simulink model "LGS_allFaultStuffDeleted"  (R2019b)
settings: Solver=FixedStepDiscrete  StartTime=0.0  StopTime=45.0  FixedStep=0.1  RelTol=1e-3
model workspace (MAT data in the model file):
  fipData : object (value not decoded)
  fipName : object (value not decoded)
  stepSize = 0.1
libraries: commrandsrc3 x16, simulink x3, LibFailureCondition x1
(part 6 of 7)

== stateflow chart LGS_allFaultStuffDeleted/Digital Part/Computing module2/GenericMonitoring9/GenericMonitoring2 ==
  state SensorValid
    entry: anomaly = false;
  state Channel1Invalid
  state SensorInvalid
    entry: anomaly = true;
  note: If at t the three channels are considered as valid and are equal, then the
      | value considered by the control software is this common value.
  state Channel2Invalid
  note: If a channel has been eliminated previously, and if at t the two remaining
      | channels are not equal, then the sensor is definitely considered as invalid.
  state Channel3Invalid
  note: If at t one channel is different from the two others for the first time (i.e.,
      | the three channels were considered as valid up to t), then this channel is
      | considered as invalid and is definitely eliminated. Only the two remaining
      | channels are considered in the future. At time t, the value considered by the
      | control software is the common value of the two remaining channels.
  (default) -> SensorValid
  SensorValid -> Channel1Invalid [order 1] : [(((Channel3&&Channel2) || ((~Channel3)&&(~Channel2))) && ((Channel1 && (~Channel2)) || ((~Channel1) && Channel2)))]
  Channel1Invalid -> SensorInvalid : [((Channel2 && (~Channel3)) || ((~Channel2) && Channel3))]
  SensorValid -> Channel2Invalid [order 2] : [(((Channel1&&Channel3) || ((~Channel1)&&(~Channel3))) && ((Channel1 && (~Channel2)) || ((~Channel1) && Channel2)))]
  SensorValid -> Channel3Invalid [order 3] : [(((Channel1&&Channel2) || ((~Channel1)&&(~Channel2))) && ((Channel1 && (~Channel3)) || ((~Channel1) && Channel3)))]
  Channel2Invalid -> SensorInvalid : [((Channel1 && (~Channel3)) || ((~Channel1) && Channel3))]
  Channel3Invalid -> SensorInvalid : [((Channel2 && (~Channel1)) || ((~Channel2) && Channel1))]
  data: Channel1 input boolean; Channel2 input boolean; Channel3 input boolean; anomaly output boolean

== stateflow chart LGS_allFaultStuffDeleted/Doors/EV close doors/EV close doors ==
  state state_EVCloseDoorsOpened
    en: EVCloseDoorsPresure_out = false;
  state state_EVCloseDoorsClose
    en: EVCloseDoorsPresure_out = false;
  state state_EVCloseDoorsClosed
    en: EVCloseDoorsPresure_out = true;
  (default) -> state_EVCloseDoorsOpened
  state_EVCloseDoorsClosed -> state_EVCloseDoorsOpened : [((~signal_in) || (~EVCloseDoorsPresure_in)) && ~fail]
  state_EVCloseDoorsOpened -> state_EVCloseDoorsClose : [(signal_in && EVCloseDoorsPresure_in && ~fail)]
  state_EVCloseDoorsClose -> state_EVCloseDoorsOpened [order 2] : [((~signal_in) || (~EVCloseDoorsPresure_in)) && ~fail]
  state_EVCloseDoorsClose -> state_EVCloseDoorsClosed [order 1] : [(signal_in && EVCloseDoorsPresure_in && ~fail)]
  data: signal_in input boolean; EVCloseDoorsPresure_in input boolean [0..1]; EVCloseDoorsPresure_out output boolean [0..1]; fail input

== stateflow chart LGS_allFaultStuffDeleted/Doors/EV open doors/EV open doors ==
  state state_EVOpenDoorsOpened
    en: EVOpenDoorsPresure_out = false;
  state state_EVOpenDoorsClose
    en: EVOpenDoorsPresure_out = false;
  state state_EVOpenDoorsClosed
    en: EVOpenDoorsPresure_out = true;
  (default) -> state_EVOpenDoorsOpened
  state_EVOpenDoorsClosed -> state_EVOpenDoorsOpened : [((~signal_in) || (~EVOpenDoorsPresure_in)) && ~fail]
  state_EVOpenDoorsOpened -> state_EVOpenDoorsClose : [(signal_in && EVOpenDoorsPresure_in && ~fail)]
  state_EVOpenDoorsClose -> state_EVOpenDoorsOpened [order 2] : [((~signal_in) || (~EVOpenDoorsPresure_in)) && ~fail]
  state_EVOpenDoorsClose -> state_EVOpenDoorsClosed [order 1] : [(signal_in && EVOpenDoorsPresure_in && ~fail)]
  data: signal_in input boolean; EVOpenDoorsPresure_in input boolean [0..1]; EVOpenDoorsPresure_out output boolean [0..1]; fail input

== stateflow chart LGS_allFaultStuffDeleted/Doors/left door zylinder/door zylinder ==
  state state_DoorZylinderClosedLocked
    en: doorZylinderOpen = false;
    en: doorZylinderLockedClosed = true;
  state state_DoorZylinderClosedLock
    en: doorZylinderOpen = false;
    en: doorZylinderLockedClosed = false;
  state state_DoorZylinderClose
    en: doorZylinderOpen = false;
    en: doorZylinderLockedClosed = false;
    en: time = int8(1);
    du: time = time - 1;
  state state_DoorZylinderClosedLockingPaused
    en: doorZylinderOpen = false;
    en: doorZylinderLockedClosed = false;
  state state_DoorZylinderClosedUnlock
    en: doorZylinderOpen = false;
    en: doorZylinderLockedClosed = false;
  state state_DoorZylinderMovingPaused
    en: doorZylinderOpen = false;
    en: doorZylinderLockedClosed = false;
  state state_DoorZylinderOpen
    en: doorZylinderOpen = false;
    en: doorZylinderLockedClosed = false;
    en: time = int8(1);
    du: time = time - 1;
  state state_DoorZylinderOpened
    en: doorZylinderOpen = true;
    en: doorZylinderLockedClosed = false;
  state state_DoorZylinderOpenedPaused
    en: doorZylinderOpen = false;
    en: doorZylinderLockedClosed = false;
  (default) -> state_DoorZylinderClosedLocked
  state_DoorZylinderClose -> state_DoorZylinderClosedLock [order 1] : [((time==0) && (~presureOpenDoor) && presureCloseDoor && (~fail))]
  state_DoorZylinderClosedLock -> state_DoorZylinderClosedLocked [order 1] : [((~presureOpenDoor) && presureCloseDoor && (~fail))]
  state_DoorZylinderClosedUnlock -> state_DoorZylinderClosedLock [order 1] : [((~presureOpenDoor) && presureCloseDoor && (~fail))]
  state_DoorZylinderClosedLock -> state_DoorZylinderClosedUnlock [order 2] : [(presureOpenDoor && (~presureCloseDoor) && (~fail))]
  state_DoorZylinderClosedLocked -> state_DoorZylinderClosedUnlock : [(presureOpenDoor && (~presureCloseDoor) && (~fail))]
  state_DoorZylinderClosedLockingPaused -> state_DoorZylinderClosedLock [order 2] : [((~presureOpenDoor) && presureCloseDoor && (~fail))]
  state_DoorZylinderClosedLock -> state_DoorZylinderClosedLockingPaused [order 3] : [(((~presureOpenDoor) && (~presureCloseDoor)) || (presureOpenDoor && presureCloseDoor) || fail)]
  state_DoorZylinderClose -> state_DoorZylinderMovingPaused [order 3] : [(((~presureOpenDoor) && (~presureCloseDoor)) || (presureOpenDoor && presureCloseDoor) || fail)]
  state_DoorZylinderOpenedPaused -> state_DoorZylinderClose [order 2] : [((~presureOpenDoor) && presureCloseDoor && (~fail))]
  state_DoorZylinderOpen -> state_DoorZylinderClose [order 2] : [((~presureOpenDoor) && presureCloseDoor && (~fail))]
  state_DoorZylinderClose -> state_DoorZylinderOpen [order 2] : [(presureOpenDoor && (~presureCloseDoor) && (~fail))]
  state_DoorZylinderMovingPaused -> state_DoorZylinderClose [order 2] : [((~presureOpenDoor) && presureCloseDoor && (~fail))]
  state_DoorZylinderOpened -> state_DoorZylinderClose [order 2] : [((~presureOpenDoor) && presureCloseDoor && (~fail))]
  state_DoorZylinderClosedLockingPaused -> state_DoorZylinderClosedUnlock [order 1] : [(presureOpenDoor && (~presureCloseDoor) && (~fail))]
  state_DoorZylinderClosedUnlock -> state_DoorZylinderClosedLockingPaused [order 2] : [(((~presureOpenDoor) && (~presureCloseDoor)) || (presureOpenDoor && presureCloseDoor) || fail)]
  state_DoorZylinderClosedUnlock -> state_DoorZylinderOpen [order 3] : [(presureOpenDoor && (~presureCloseDoor) && (~fail))]
  state_DoorZylinderOpen -> state_DoorZylinderMovingPaused [order 3] : [(((~presureOpenDoor) && (~presureCloseDoor)) || (presureOpenDoor && presureCloseDoor) || fail)]
  state_DoorZylinderMovingPaused -> state_DoorZylinderOpen [order 1] : [(presureOpenDoor && (~presureCloseDoor) && (~fail))]
  state_DoorZylinderOpen -> state_DoorZylinderOpened [order 1] : [((time==0) && presureOpenDoor && (~presureCloseDoor) && (~fail))]
  state_DoorZylinderOpened -> state_DoorZylinderOpenedPaused [order 1] : [(((~presureOpenDoor) && (~presureCloseDoor) && (~fail)) || (presureOpenDoor && presureCloseDoor && (~fail)))]
  state_DoorZylinderOpenedPaused -> state_DoorZylinderOpened [order 1] : [(presureOpenDoor && (~presureCloseDoor) && (~fail))]
  data: presureOpenDoor input boolean [0..1]; presureCloseDoor input boolean [0..1]; time local int8 [0..1]; doorZylinderLockedClosed output boolean; doorZylinderOpen output boolean; fail input boolean

== stateflow chart LGS_allFaultStuffDeleted/Doors/right door zylinder/door zylinder ==
  state state_DoorZylinderClosedLocked
    en: doorZylinderOpen = false;
    en: doorZylinderLockedClosed = true;
  state state_DoorZylinderClosedLock
    en: doorZylinderOpen = false;
    en: doorZylinderLockedClosed = false;
  state state_DoorZylinderClose
    en: doorZylinderOpen = false;
    en: doorZylinderLockedClosed = false;
    en: time = int8(1);
    du: time = time - 1;
  state state_DoorZylinderClosedLockingPaused
    en: doorZylinderOpen = false;
    en: doorZylinderLockedClosed = false;
  state state_DoorZylinderClosedUnlock
    en: doorZylinderOpen = false;
    en: doorZylinderLockedClosed = false;
  state state_DoorZylinderMovingPaused
    en: doorZylinderOpen = false;
    en: doorZylinderLockedClosed = false;
  state state_DoorZylinderOpen
    en: doorZylinderOpen = false;
    en: doorZylinderLockedClosed = false;
    en: time = int8(1);
    du: time = time - 1;
  state state_DoorZylinderOpened
    en: doorZylinderOpen = true;
    en: doorZylinderLockedClosed = false;
  state state_DoorZylinderOpenedPaused
    en: doorZylinderOpen = false;
    en: doorZylinderLockedClosed = false;
  (default) -> state_DoorZylinderClosedLocked
  state_DoorZylinderClose -> state_DoorZylinderClosedLock [order 1] : [((time==0) && (~presureOpenDoor) && presureCloseDoor && (~fail))]
  state_DoorZylinderClosedLock -> state_DoorZylinderClosedLocked [order 1] : [((~presureOpenDoor) && presureCloseDoor && (~fail))]
  state_DoorZylinderClosedUnlock -> state_DoorZylinderClosedLock [order 1] : [((~presureOpenDoor) && presureCloseDoor && (~fail))]
  state_DoorZylinderClosedLock -> state_DoorZylinderClosedUnlock [order 2] : [(presureOpenDoor && (~presureCloseDoor) && (~fail))]
  state_DoorZylinderClosedLocked -> state_DoorZylinderClosedUnlock : [(presureOpenDoor && (~presureCloseDoor) && (~fail))]
  state_DoorZylinderClosedLockingPaused -> state_DoorZylinderClosedLock [order 2] : [((~presureOpenDoor) && presureCloseDoor && (~fail))]
  state_DoorZylinderClosedLock -> state_DoorZylinderClosedLockingPaused [order 3] : [(((~presureOpenDoor) && (~presureCloseDoor)) || (presureOpenDoor && presureCloseDoor) || fail)]
  state_DoorZylinderClose -> state_DoorZylinderMovingPaused [order 3] : [(((~presureOpenDoor) && (~presureCloseDoor)) || (presureOpenDoor && presureCloseDoor) || fail)]
  state_DoorZylinderOpenedPaused -> state_DoorZylinderClose [order 2] : [((~presureOpenDoor) && presureCloseDoor && (~fail))]
  state_DoorZylinderOpen -> state_DoorZylinderClose [order 2] : [((~presureOpenDoor) && presureCloseDoor && (~fail))]
  state_DoorZylinderClose -> state_DoorZylinderOpen [order 2] : [(presureOpenDoor && (~presureCloseDoor) && (~fail))]
  state_DoorZylinderMovingPaused -> state_DoorZylinderClose [order 2] : [((~presureOpenDoor) && presureCloseDoor && (~fail))]
  state_DoorZylinderOpened -> state_DoorZylinderClose [order 2] : [((~presureOpenDoor) && presureCloseDoor && (~fail))]
  state_DoorZylinderClosedLockingPaused -> state_DoorZylinderClosedUnlock [order 1] : [(presureOpenDoor && (~presureCloseDoor) && (~fail))]
  state_DoorZylinderClosedUnlock -> state_DoorZylinderClosedLockingPaused [order 2] : [(((~presureOpenDoor) && (~presureCloseDoor)) || (presureOpenDoor && presureCloseDoor) || fail)]
  state_DoorZylinderClosedUnlock -> state_DoorZylinderOpen [order 3] : [(presureOpenDoor && (~presureCloseDoor) && (~fail))]
  state_DoorZylinderOpen -> state_DoorZylinderMovingPaused [order 3] : [(((~presureOpenDoor) && (~presureCloseDoor)) || (presureOpenDoor && presureCloseDoor) || fail)]
  state_DoorZylinderMovingPaused -> state_DoorZylinderOpen [order 1] : [(presureOpenDoor && (~presureCloseDoor) && (~fail))]
  state_DoorZylinderOpen -> state_DoorZylinderOpened [order 1] : [((time==0) && presureOpenDoor && (~presureCloseDoor) && (~fail))]
  state_DoorZylinderOpened -> state_DoorZylinderOpenedPaused [order 1] : [(((~presureOpenDoor) && (~presureCloseDoor) && (~fail)) || (presureOpenDoor && presureCloseDoor && (~fail)))]
  state_DoorZylinderOpenedPaused -> state_DoorZylinderOpened [order 1] : [(presureOpenDoor && (~presureCloseDoor) && (~fail))]
  data: presureOpenDoor input boolean [0..1]; presureCloseDoor input boolean [0..1]; time local int8 [0..1]; doorZylinderLockedClosed output boolean; doorZylinderOpen output boolean; fail input boolean

== stateflow chart LGS_allFaultStuffDeleted/Doors/front door zylinder/door cylinder ==
  state state_DoorZylinderClosedLocked
    en: doorZylinderOpen = false;
    en: doorZylinderLockedClosed = true;
  state state_DoorZylinderClosedLock
    en: doorZylinderOpen = false;
    en: doorZylinderLockedClosed = false;
  state state_DoorZylinderClose
    en: doorZylinderOpen = false;
    en: doorZylinderLockedClosed = false;
    en: time = int8(1);
    du: time = time - 1;
  state state_DoorZylinderClosedLockingPaused
    en: doorZylinderOpen = false;
    en: doorZylinderLockedClosed = false;
  state state_DoorZylinderClosedUnlock
    en: doorZylinderOpen = false;
    en: doorZylinderLockedClosed = false;
  state state_DoorZylinderMovingPaused
    en: doorZylinderOpen = false;
    en: doorZylinderLockedClosed = false;
  state state_DoorZylinderOpen
    en: doorZylinderOpen = false;
    en: doorZylinderLockedClosed = false;
    en: time = int8(1);
    du: time = time - 1;
  state state_DoorZylinderOpened
    en: doorZylinderOpen = true;
    en: doorZylinderLockedClosed = false;
  state state_DoorZylinderOpenedPaused
    en: doorZylinderOpen = false;
    en: doorZylinderLockedClosed = false;
  (default) -> state_DoorZylinderClosedLocked
  state_DoorZylinderClose -> state_DoorZylinderClosedLock [order 1] : [((time==0) && (~presureOpenDoor) && presureCloseDoor && (~fail))]
  state_DoorZylinderClosedLock -> state_DoorZylinderClosedLocked [order 1] : [((~presureOpenDoor) && presureCloseDoor && (~fail))]
  state_DoorZylinderClosedUnlock -> state_DoorZylinderClosedLock [order 1] : [((~presureOpenDoor) && presureCloseDoor && (~fail))]
  state_DoorZylinderClosedLock -> state_DoorZylinderClosedUnlock [order 2] : [(presureOpenDoor && (~presureCloseDoor) && (~fail))]
  state_DoorZylinderClosedLocked -> state_DoorZylinderClosedUnlock : [(presureOpenDoor && (~presureCloseDoor) && (~fail))]
  state_DoorZylinderClosedLockingPaused -> state_DoorZylinderClosedLock [order 2] : [((~presureOpenDoor) && presureCloseDoor && (~fail))]
  state_DoorZylinderClosedLock -> state_DoorZylinderClosedLockingPaused [order 3] : [(((~presureOpenDoor) && (~presureCloseDoor)) || (presureOpenDoor && presureCloseDoor) || fail)]
  state_DoorZylinderClose -> state_DoorZylinderMovingPaused [order 3] : [(((~presureOpenDoor) && (~presureCloseDoor)) || (presureOpenDoor && presureCloseDoor) || fail)]
  state_DoorZylinderOpenedPaused -> state_DoorZylinderClose [order 2] : [((~presureOpenDoor) && presureCloseDoor && (~fail))]
  state_DoorZylinderOpen -> state_DoorZylinderClose [order 2] : [((~presureOpenDoor) && presureCloseDoor && (~fail))]
  state_DoorZylinderClose -> state_DoorZylinderOpen [order 2] : [(presureOpenDoor && (~presureCloseDoor) && (~fail))]
  state_DoorZylinderMovingPaused -> state_DoorZylinderClose [order 2] : [((~presureOpenDoor) && presureCloseDoor && (~fail))]
  state_DoorZylinderOpened -> state_DoorZylinderClose [order 2] : [((~presureOpenDoor) && presureCloseDoor && (~fail))]
  state_DoorZylinderClosedLockingPaused -> state_DoorZylinderClosedUnlock [order 1] : [(presureOpenDoor && (~presureCloseDoor) && (~fail))]
  state_DoorZylinderClosedUnlock -> state_DoorZylinderClosedLockingPaused [order 2] : [(((~presureOpenDoor) && (~presureCloseDoor)) || (presureOpenDoor && presureCloseDoor) || fail)]
  state_DoorZylinderClosedUnlock -> state_DoorZylinderOpen [order 3] : [(presureOpenDoor && (~presureCloseDoor) && (~fail))]
  state_DoorZylinderOpen -> state_DoorZylinderMovingPaused [order 3] : [(((~presureOpenDoor) && (~presureCloseDoor)) || (presureOpenDoor && presureCloseDoor) || fail)]
  state_DoorZylinderMovingPaused -> state_DoorZylinderOpen [order 1] : [(presureOpenDoor && (~presureCloseDoor) && (~fail))]
  state_DoorZylinderOpen -> state_DoorZylinderOpened [order 1] : [((time==0) && presureOpenDoor && (~presureCloseDoor) && (~fail))]
  state_DoorZylinderOpened -> state_DoorZylinderOpenedPaused [order 1] : [(((~presureOpenDoor) && (~presureCloseDoor) && (~fail)) || (presureOpenDoor && presureCloseDoor && (~fail)))]
  state_DoorZylinderOpenedPaused -> state_DoorZylinderOpened [order 1] : [(presureOpenDoor && (~presureCloseDoor) && (~fail))]
  data: presureOpenDoor input boolean [0..1]; presureCloseDoor input boolean [0..1]; time local int8 [0..1]; doorZylinderLockedClosed output boolean; doorZylinderOpen output boolean; fail input boolean

== stateflow chart LGS_allFaultStuffDeleted/Gears/EV extend gear/EV extend gear ==
  state state_EVExtendGearOpened
    en: EVExtendGearPresure_out = false;
  state state_EVExtendGearClose
    en: EVExtendGearPresure_out = false;
  state state_EVExtendGearClosed
    en: EVExtendGearPresure_out = true;
  (default) -> state_EVExtendGearOpened
  state_EVExtendGearClosed -> state_EVExtendGearOpened : [((~signal_in) || (~EVExtendGearPresure_in)) && ~fail]
  state_EVExtendGearOpened -> state_EVExtendGearClose : [(signal_in && EVExtendGearPresure_in && ~fail)]
  state_EVExtendGearClose -> state_EVExtendGearOpened [order 2] : [((~signal_in) || (~EVExtendGearPresure_in)) && ~fail]
  state_EVExtendGearClose -> state_EVExtendGearClosed [order 1] : [(signal_in && EVExtendGearPresure_in && ~fail)]
  data: signal_in input boolean; EVExtendGearPresure_in input boolean [0..1]; EVExtendGearPresure_out output boolean [0..1]; fail input

== stateflow chart LGS_allFaultStuffDeleted/Gears/EV retract gear/EV retract gear ==
  state state_EVRetractGearOpened
    en: EVRetractGearPresure_out = false;
  state state_EVRetractGearClose
    en: EVRetractGearPresure_out = false;
  state state_EVRetractGearClosed
    en: EVRetractGearPresure_out = true;
  (default) -> state_EVRetractGearOpened
  state_EVRetractGearClosed -> state_EVRetractGearOpened : [((~signal_in) || (~EVRetractGearPresure_in)) && ~fail]
  state_EVRetractGearOpened -> state_EVRetractGearClose : [(signal_in && EVRetractGearPresure_in && ~fail)]
  state_EVRetractGearClose -> state_EVRetractGearOpened [order 2] : [((~signal_in) || (~EVRetractGearPresure_in)) && ~fail]
  state_EVRetractGearClose -> state_EVRetractGearClosed [order 1] : [(signal_in && EVRetractGearPresure_in && ~fail)]
  data: signal_in input boolean; EVRetractGearPresure_in input boolean [0..1]; EVRetractGearPresure_out output boolean [0..1]; fail input

== stateflow chart LGS_allFaultStuffDeleted/Gears/front gear cylinder/gear zylinder ==
  state state_GearZylinderRetractedLock
    en: gearLockedRetracted = false;
    en: gearLockedExtended = false;
  state state_GearZylinderRetractedLocked
    en: gearLockedRetracted = true;
    en: gearLockedExtended = false;
  state state_GearZylinderRetract
    en: gearLockedRetracted = false;
    en: gearLockedExtended = false;
    en: time = int8(1);
    du: time = time - 1;
  state state_GearZylinderRetractedPaused
    en: gearLockedRetracted = false;
    en: gearLockedExtended = false;
  state state_GearZylinderRetractedUnlock
    en: gearLockedRetracted = false;
    en: gearLockedExtended = false;
  state state_GearZylinderMovingPaused
    en: gearLockedRetracted = false;
    en: gearLockedExtended = false;
  state state_GearZylinderExtendedUnlock
    en: gearLockedRetracted = false;
    en: gearLockedExtended = false;
  state state_init
    en: gearLockedRetracted = false;
    en: gearLockedExtended = false;
  state state_GearZylinderExtendedPaused
    en: gearLockedRetracted = false;
    en: gearLockedExtended = false;
  state state_GearZylinderExtend
    en: gearLockedRetracted = false;
    en: gearLockedExtended = false;
    en: time = int8(1);
    du: time = time - 1;
  state state_GearZylinderExtendedLock
    en: gearLockedRetracted = false;
    en: gearLockedExtended = false;
  state state_GearZylinderExtendedLocked
    en: gearLockedRetracted = false;
    en: gearLockedExtended = true;
  state_GearZylinderRetractedLock -> state_GearZylinderRetractedLocked [order 1] : [(presureRetractGear && (~presureExtendGear) && (~fail))]
  state_GearZylinderRetract -> state_GearZylinderRetractedLock [order 1] : [((time==0) && presureRetractGear && (~presureExtendGear) && (~fail))]
  state_init -> state_GearZylinderRetractedLocked [order 1] : [(initHandleState)]
  state_GearZylinderRetractedLock -> state_GearZylinderRetractedUnlock [order 3] : [((~presureRetractGear) && presureExtendGear && (~fail))]
  state_GearZylinderRetractedUnlock -> state_GearZylinderRetractedLock [order 2] : [(presureRetractGear && (~presureExtendGear) && (~fail))]
  state_GearZylinderRetractedLocked -> state_GearZylinderRetractedUnlock : [((~presureRetractGear) && presureExtendGear && (~fail))]
  state_GearZylinderRetractedLock -> state_GearZylinderRetractedPaused [order 2] : [(((~presureRetractGear) && (~presureExtendGear)) || (presureRetractGear && presureExtendGear) || fail)]
  state_GearZylinderRetractedPaused -> state_GearZylinderRetractedLock [order 2] : [(presureRetractGear && (~presureExtendGear) && (~fail))]
  state_GearZylinderExtendedUnlock -> state_GearZylinderRetract [order 1] : [(presureRetractGear && (~presureExtendGear) && (~fail))]
  state_GearZylinderExtend -> state_GearZylinderRetract [order 2] : [(presureRetractGear && (~presureExtendGear) && (~fail))]
  state_GearZylinderRetract -> state_GearZylinderExtend [order 2] : [((~presureRetractGear) && presureExtendGear && (~fail))]
  state_GearZylinderMovingPaused -> state_GearZylinderRetract [order 2] : [(presureRetractGear && (~presureExtendGear) && (~fail))]
  state_GearZylinderRetract -> state_GearZylinderMovingPaused [order 3] : [(((~presureRetractGear) && (~presureExtendGear)) || (presureRetractGear && presureExtendGear) || fail)]
  state_GearZylinderRetractedPaused -> state_GearZylinderRetractedUnlock [order 1] : [((~presureRetractGear) && presureExtendGear && (~fail))]
  state_GearZylinderRetractedUnlock -> state_GearZylinderRetractedPaused [order 3] : [(((~presureRetractGear) && (~presureExtendGear)) || (presureRetractGear && presureExtendGear) || fail)]
  state_GearZylinderRetractedUnlock -> state_GearZylinderExtend [order 1] : [((~presureRetractGear) && presureExtendGear && (~fail))]
  state_GearZylinderExtendedUnlock -> state_GearZylinderExtendedPaused [order 3] : [(((~presureRetractGear) && (~presureExtendGear)) || (presureRetractGear && presureExtendGear) || fail)]
  (default) -> state_init
  state_GearZylinderMovingPaused -> state_GearZylinderExtend [order 1] : [((~presureRetractGear) && presureExtendGear && (~fail))]
  state_GearZylinderExtend -> state_GearZylinderMovingPaused [order 3] : [(((~presureRetractGear) && (~presureExtendGear)) || (presureRetractGear && presureExtendGear) || fail)]
  state_GearZylinderExtendedPaused -> state_GearZylinderExtendedUnlock [order 2] : [(presureRetractGear && (~presureExtendGear) && (~fail))]
  state_GearZylinderExtendedUnlock -> state_GearZylinderExtendedLock [order 2] : [((~presureRetractGear) && presureExtendGear && (~fail))]
  state_GearZylinderExtendedLock -> state_GearZylinderExtendedUnlock [order 2] : [(presureRetractGear && (~presureExtendGear) && (~fail))]
  state_GearZylinderExtendedLocked -> state_GearZylinderExtendedUnlock : [(presureRetractGear && (~presureExtendGear) && (~fail))]
  state_init -> state_GearZylinderExtendedLocked [order 2] : [(~initHandleState)]
  state_GearZylinderExtendedLock -> state_GearZylinderExtendedPaused [order 3] : [(((~presureRetractGear) && (~presureExtendGear)) || (presureRetractGear && presureExtendGear) || fail)]
  state_GearZylinderExtendedPaused -> state_GearZylinderExtendedLock [order 1] : [((~presureRetractGear) && presureExtendGear && (~fail))]
  state_GearZylinderExtend -> state_GearZylinderExtendedLock [order 1] : [((time==0) && (~presureRetractGear) && presureExtendGear && (~fail))]
  state_GearZylinderExtendedLock -> state_GearZylinderExtendedLocked [order 1] : [((~presureRetractGear) && presureExtendGear && (~fail))]
  data: presureExtendGear input boolean [0..1]; presureRetractGear input boolean [0..1]; gearLockedExtended output boolean [0..1]; gearLockedRetracted output boolean [0..1]; time local int8 [0..1]; fail input boolean; initHandleState input boolean

== stateflow chart LGS_allFaultStuffDeleted/Gears/left gear cylinder/gear zylinder ==
  state state_GearZylinderRetractedLock
    en: gearLockedRetracted = false;
    en: gearLockedExtended = false;
  state state_GearZylinderRetractedLocked
    en: gearLockedRetracted = true;
    en: gearLockedExtended = false;
  state state_GearZylinderRetract
    en: gearLockedRetracted = false;
    en: gearLockedExtended = false;
    en: time = int8(1);
    du: time = time - 1;
  state state_GearZylinderRetractedPaused
    en: gearLockedRetracted = false;
    en: gearLockedExtended = false;
  state state_GearZylinderRetractedUnlock
    en: gearLockedRetracted = false;
    en: gearLockedExtended = false;
  state state_GearZylinderMovingPaused
    en: gearLockedRetracted = false;
    en: gearLockedExtended = false;
  state state_GearZylinderExtendedUnlock
    en: gearLockedRetracted = false;
    en: gearLockedExtended = false;
  state state_init
    en: gearLockedRetracted = false;
    en: gearLockedExtended = false;
  state state_GearZylinderExtendedPaused
    en: gearLockedRetracted = false;
    en: gearLockedExtended = false;
  state state_GearZylinderExtend
    en: gearLockedRetracted = false;
    en: gearLockedExtended = false;
    en: time = int8(1);
    du: time = time - 1;
  state state_GearZylinderExtendedLock
    en: gearLockedRetracted = false;
    en: gearLockedExtended = false;
  state state_GearZylinderExtendedLocked
    en: gearLockedRetracted = false;
    en: gearLockedExtended = true;
  state_GearZylinderRetractedLock -> state_GearZylinderRetractedLocked [order 1] : [(presureRetractGear && (~presureExtendGear) && (~fail))]
  state_GearZylinderRetract -> state_GearZylinderRetractedLock [order 1] : [((time==0) && presureRetractGear && (~presureExtendGear) && (~fail))]
  state_init -> state_GearZylinderRetractedLocked [order 1] : [(initHandleState)]
  state_GearZylinderRetractedLock -> state_GearZylinderRetractedUnlock [order 3] : [((~presureRetractGear) && presureExtendGear && (~fail))]
  state_GearZylinderRetractedUnlock -> state_GearZylinderRetractedLock [order 2] : [(presureRetractGear && (~presureExtendGear) && (~fail))]
  state_GearZylinderRetractedLocked -> state_GearZylinderRetractedUnlock : [((~presureRetractGear) && presureExtendGear && (~fail))]
  state_GearZylinderRetractedLock -> state_GearZylinderRetractedPaused [order 2] : [(((~presureRetractGear) && (~presureExtendGear)) || (presureRetractGear && presureExtendGear) || fail)]
  state_GearZylinderRetractedPaused -> state_GearZylinderRetractedLock [order 2] : [(presureRetractGear && (~presureExtendGear) && (~fail))]
  state_GearZylinderExtendedUnlock -> state_GearZylinderRetract [order 1] : [(presureRetractGear && (~presureExtendGear) && (~fail))]
  state_GearZylinderExtend -> state_GearZylinderRetract [order 2] : [(presureRetractGear && (~presureExtendGear) && (~fail))]
  state_GearZylinderRetract -> state_GearZylinderExtend [order 2] : [((~presureRetractGear) && presureExtendGear && (~fail))]
  state_GearZylinderMovingPaused -> state_GearZylinderRetract [order 2] : [(presureRetractGear && (~presureExtendGear) && (~fail))]
  state_GearZylinderRetract -> state_GearZylinderMovingPaused [order 3] : [(((~presureRetractGear) && (~presureExtendGear)) || (presureRetractGear && presureExtendGear) || fail)]
  state_GearZylinderRetractedPaused -> state_GearZylinderRetractedUnlock [order 1] : [((~presureRetractGear) && presureExtendGear && (~fail))]
  state_GearZylinderRetractedUnlock -> state_GearZylinderRetractedPaused [order 3] : [(((~presureRetractGear) && (~presureExtendGear)) || (presureRetractGear && presureExtendGear) || fail)]
  state_GearZylinderRetractedUnlock -> state_GearZylinderExtend [order 1] : [((~presureRetractGear) && presureExtendGear && (~fail))]
  state_GearZylinderExtendedUnlock -> state_GearZylinderExtendedPaused [order 3] : [(((~presureRetractGear) && (~presureExtendGear)) || (presureRetractGear && presureExtendGear) || fail)]
  (default) -> state_init
  state_GearZylinderMovingPaused -> state_GearZylinderExtend [order 1] : [((~presureRetractGear) && presureExtendGear && (~fail))]
  state_GearZylinderExtend -> state_GearZylinderMovingPaused [order 3] : [(((~presureRetractGear) && (~presureExtendGear)) || (presureRetractGear && presureExtendGear) || fail)]
  state_GearZylinderExtendedPaused -> state_GearZylinderExtendedUnlock [order 2] : [(presureRetractGear && (~presureExtendGear) && (~fail))]
  state_GearZylinderExtendedUnlock -> state_GearZylinderExtendedLock [order 2] : [((~presureRetractGear) && presureExtendGear && (~fail))]
  state_GearZylinderExtendedLock -> state_GearZylinderExtendedUnlock [order 2] : [(presureRetractGear && (~presureExtendGear) && (~fail))]
  state_GearZylinderExtendedLocked -> state_GearZylinderExtendedUnlock : [(presureRetractGear && (~presureExtendGear) && (~fail))]
  state_init -> state_GearZylinderExtendedLocked [order 2] : [(~initHandleState)]
  state_GearZylinderExtendedLock -> state_GearZylinderExtendedPaused [order 3] : [(((~presureRetractGear) && (~presureExtendGear)) || (presureRetractGear && presureExtendGear) || fail)]
  state_GearZylinderExtendedPaused -> state_GearZylinderExtendedLock [order 1] : [((~presureRetractGear) && presureExtendGear && (~fail))]
  state_GearZylinderExtend -> state_GearZylinderExtendedLock [order 1] : [((time==0) && (~presureRetractGear) && presureExtendGear && (~fail))]
  state_GearZylinderExtendedLock -> state_GearZylinderExtendedLocked [order 1] : [((~presureRetractGear) && presureExtendGear && (~fail))]
  data: presureExtendGear input boolean [0..1]; presureRetractGear input boolean [0..1]; gearLockedExtended output boolean [0..1]; gearLockedRetracted output boolean [0..1]; time local int8 [0..1]; fail input boolean; initHandleState input boolean

== stateflow chart LGS_allFaultStuffDeleted/Gears/right gear cylinder/gear zylinder ==
  state state_GearZylinderRetractedLock
    en: gearLockedRetracted = false;
    en: gearLockedExtended = false;
  state state_GearZylinderRetractedLocked
    en: gearLockedRetracted = true;
    en: gearLockedExtended = false;
  state state_GearZylinderRetract
    en: gearLockedRetracted = false;
    en: gearLockedExtended = false;
    en: time = int8(1);
    du: time = time - 1;
  state state_GearZylinderRetractedPaused
    en: gearLockedRetracted = false;
    en: gearLockedExtended = false;
  state state_GearZylinderRetractedUnlock
    en: gearLockedRetracted = false;
    en: gearLockedExtended = false;
  state state_GearZylinderMovingPaused
    en: gearLockedRetracted = false;
    en: gearLockedExtended = false;
  state state_GearZylinderExtendedUnlock
    en: gearLockedRetracted = false;
    en: gearLockedExtended = false;
  state state_init
    en: gearLockedRetracted = false;
    en: gearLockedExtended = false;
  state state_GearZylinderExtendedPaused
    en: gearLockedRetracted = false;
    en: gearLockedExtended = false;
  state state_GearZylinderExtend
    en: gearLockedRetracted = false;
    en: gearLockedExtended = false;
    en: time = int8(1);
    du: time = time - 1;
  state state_GearZylinderExtendedLock
    en: gearLockedRetracted = false;
    en: gearLockedExtended = false;
  state state_GearZylinderExtendedLocked
    en: gearLockedRetracted = false;
    en: gearLockedExtended = true;
  state_GearZylinderRetractedLock -> state_GearZylinderRetractedLocked [order 1] : [(presureRetractGear && (~presureExtendGear) && (~fail))]
  state_GearZylinderRetract -> state_GearZylinderRetractedLock [order 1] : [((time==0) && presureRetractGear && (~presureExtendGear) && (~fail))]
  state_init -> state_GearZylinderRetractedLocked [order 1] : [(initHandleState)]
  state_GearZylinderRetractedLock -> state_GearZylinderRetractedUnlock [order 3] : [((~presureRetractGear) && presureExtendGear && (~fail))]
  state_GearZylinderRetractedUnlock -> state_GearZylinderRetractedLock [order 2] : [(presureRetractGear && (~presureExtendGear) && (~fail))]
  state_GearZylinderRetractedLocked -> state_GearZylinderRetractedUnlock : [((~presureRetractGear) && presureExtendGear && (~fail))]
  state_GearZylinderRetractedLock -> state_GearZylinderRetractedPaused [order 2] : [(((~presureRetractGear) && (~presureExtendGear)) || (presureRetractGear && presureExtendGear) || fail)]
  state_GearZylinderRetractedPaused -> state_GearZylinderRetractedLock [order 2] : [(presureRetractGear && (~presureExtendGear) && (~fail))]
  state_GearZylinderExtendedUnlock -> state_GearZylinderRetract [order 1] : [(presureRetractGear && (~presureExtendGear) && (~fail))]
  state_GearZylinderExtend -> state_GearZylinderRetract [order 2] : [(presureRetractGear && (~presureExtendGear) && (~fail))]
  state_GearZylinderRetract -> state_GearZylinderExtend [order 2] : [((~presureRetractGear) && presureExtendGear && (~fail))]
  state_GearZylinderMovingPaused -> state_GearZylinderRetract [order 2] : [(presureRetractGear && (~presureExtendGear) && (~fail))]
  state_GearZylinderRetract -> state_GearZylinderMovingPaused [order 3] : [(((~presureRetractGear) && (~presureExtendGear)) || (presureRetractGear && presureExtendGear) || fail)]
  state_GearZylinderRetractedPaused -> state_GearZylinderRetractedUnlock [order 1] : [((~presureRetractGear) && presureExtendGear && (~fail))]
  state_GearZylinderRetractedUnlock -> state_GearZylinderRetractedPaused [order 3] : [(((~presureRetractGear) && (~presureExtendGear)) || (presureRetractGear && presureExtendGear) || fail)]
  state_GearZylinderRetractedUnlock -> state_GearZylinderExtend [order 1] : [((~presureRetractGear) && presureExtendGear && (~fail))]
  state_GearZylinderExtendedUnlock -> state_GearZylinderExtendedPaused [order 3] : [(((~presureRetractGear) && (~presureExtendGear)) || (presureRetractGear && presureExtendGear) || fail)]
  (default) -> state_init
  state_GearZylinderMovingPaused -> state_GearZylinderExtend [order 1] : [((~presureRetractGear) && presureExtendGear && (~fail))]
  state_GearZylinderExtend -> state_GearZylinderMovingPaused [order 3] : [(((~presureRetractGear) && (~presureExtendGear)) || (presureRetractGear && presureExtendGear) || fail)]
  state_GearZylinderExtendedPaused -> state_GearZylinderExtendedUnlock [order 2] : [(presureRetractGear && (~presureExtendGear) && (~fail))]
  state_GearZylinderExtendedUnlock -> state_GearZylinderExtendedLock [order 2] : [((~presureRetractGear) && presureExtendGear && (~fail))]
  state_GearZylinderExtendedLock -> state_GearZylinderExtendedUnlock [order 2] : [(presureRetractGear && (~presureExtendGear) && (~fail))]
  state_GearZylinderExtendedLocked -> state_GearZylinderExtendedUnlock : [(presureRetractGear && (~presureExtendGear) && (~fail))]
  state_init -> state_GearZylinderExtendedLocked [order 2] : [(~initHandleState)]
  state_GearZylinderExtendedLock -> state_GearZylinderExtendedPaused [order 3] : [(((~presureRetractGear) && (~presureExtendGear)) || (presureRetractGear && presureExtendGear) || fail)]
  state_GearZylinderExtendedPaused -> state_GearZylinderExtendedLock [order 1] : [((~presureRetractGear) && presureExtendGear && (~fail))]
  state_GearZylinderExtend -> state_GearZylinderExtendedLock [order 1] : [((time==0) && (~presureRetractGear) && presureExtendGear && (~fail))]
  state_GearZylinderExtendedLock -> state_GearZylinderExtendedLocked [order 1] : [((~presureRetractGear) && presureExtendGear && (~fail))]
  data: presureExtendGear input boolean [0..1]; presureRetractGear input boolean [0..1]; gearLockedExtended output boolean [0..1]; gearLockedRetracted output boolean [0..1]; time local int8 [0..1]; fail input boolean; initHandleState input boolean

== stateflow chart LGS_allFaultStuffDeleted/Digital Part/Computing module2/OutgoingSequence ==
  state Idle
    entry: GeneralValve = false;
    entry: OpenDoorValve = false;
    entry: GearExtensionValve = false;
    entry: CloseDoorValve = false;
    entry: stateNumber = int8(0);
  state CloseGeneralValve
    entry: GeneralValve = false;
    entry: stateNumber = int8(6);
  state InterruptDetected
    entry: GeneralValve = true;
  state StopStimulatingCloseDoorValve
    entry: CloseDoorValve = false;
    entry: stateNumber = int8(5);
  state stimulateGeneralValve
    entry: GeneralValve = true;
    entry: stateNumber = int8(1);
  state Interruption
    entry: GearExtensionValve = false;
  state StimulateOpenDoorValve
    entry: OpenDoorValve = true;
    entry: CloseDoorValve = false;
    entry: stateNumber = int8(2);
  state StopGEVandODVstartCDV
    entry: GearExtensionValve = false;
    entry: OpenDoorValve = false;
    entry: CloseDoorValve = true;
    entry: stateNumber = int8(4);
  state StimulateGearExtensionValve
    entry: GearExtensionValve = true;
    entry: stateNumber = int8(3);
  (default) -> Idle
  CloseGeneralValve -> Idle [order 1] : [(~RetractionInterruption)]
  InterruptDetected -> CloseGeneralValve [order 2] : [(InterruptStateNo == 1)]
  Idle -> InterruptDetected [order 2] : [((InterruptStateNo ~=0) && (StartOutgoingSequence))]
  CloseGeneralValve -> Interruption [order 2] : [(RetractionInterruption)]
  Interruption -> Idle
  StopStimulatingCloseDoorValve -> CloseGeneralValve [order 1] : [(~RetractionInterruption)]
  Idle -> stimulateGeneralValve [order 1] : [((((StartOutgoingSequence) && (AllGearsLockedUp)) && (AllDoorsLockedClosed)) && (InterruptStateNo == 0))]
  InterruptDetected -> stimulateGeneralValve [order 4] : [(InterruptStateNo == 6)]
  InterruptDetected -> StimulateOpenDoorValve [order 5] : [((InterruptStateNo == 4) || (InterruptStateNo == 5))]
  InterruptDetected -> StopGEVandODVstartCDV [order 3] : [(InterruptStateNo == 2)]
  stimulateGeneralValve -> Interruption [order 1] : [(RetractionInterruption)]
  InterruptDetected -> StimulateGearExtensionValve [order 1] : [(InterruptStateNo == 3)]
  stimulateGeneralValve -> StimulateOpenDoorValve [order 2] : [(~RetractionInterruption)]
  StopStimulatingCloseDoorValve -> Interruption [order 2] : [(RetractionInterruption)]
  StopGEVandODVstartCDV -> StopStimulatingCloseDoorValve [order 1] : [((AllDoorsLockedClosed) && (~RetractionInterruption))]
  StimulateOpenDoorValve -> Interruption [order 2] : [(RetractionInterruption)]
  StimulateGearExtensionValve -> Interruption [order 2] : [(RetractionInterruption)]
  StopGEVandODVstartCDV -> Interruption [order 2] : [(RetractionInterruption)]
  StimulateOpenDoorValve -> StimulateGearExtensionValve [order 1] : [((AllDoorsOpened) && (~RetractionInterruption))]
  StimulateGearExtensionValve -> StopGEVandODVstartCDV [order 1] : [((AllGearsLockedDown) && (~RetractionInterruption))]
  data: StartOutgoingSequence input boolean; GeneralValve output boolean; OpenDoorValve output boolean; AllDoorsOpened input boolean; AllDoorsLockedClosed input boolean; AllGearsLockedDown input boolean; CloseDoorValve output boolean; GearExtensionValve output boolean; AllGearsLockedUp input boolean; stateNumber output int8 [0..6]; RetractionInterruption input boolean; InterruptStateNo input int8 [0..6]

== stateflow chart LGS_allFaultStuffDeleted/Digital Part/Computing module2/PressureSensorMonitoring ==
  state Idle
    entry: anomaly = false;
  state UnpressurizeCircuit
    entry: time = int8(9);
    during: time = time -1;
  note: If the hydraulic circuit is still pressurized 10 seconds after the general electrovalve has been stopped, then an anomaly is detected in the hydraulic circuit.
  state CounterOrder1
  state PressurizeCircuit
    entry: time = int8(1);
    during: time = time - 1;
  state CounterOrder0
  state CircuitPressurized
  note: If the hydraulic circuit is still unpressurized 2 seconds after the general electro-valve has been stimulated, then an anomaly is detected in the hydraulic circuit.
  state Anomaly
    entry: anomaly = true;
  (default) -> Idle
  UnpressurizeCircuit -> Idle [order 2] : [((time == 0) && (~PressureSensor))]
  Idle -> PressurizeCircuit : [(GeneralValve)]
  UnpressurizeCircuit -> CounterOrder1 [order 3] : [(GeneralValve)]
  CounterOrder1 -> PressurizeCircuit
  CounterOrder0 -> UnpressurizeCircuit
  CircuitPressurized -> UnpressurizeCircuit : [(~GeneralValve)]
  UnpressurizeCircuit -> Anomaly [order 1] : [((time == 0) && (PressureSensor))]
  PressurizeCircuit -> CounterOrder0 [order 3] : [(~GeneralValve)]
  PressurizeCircuit -> CircuitPressurized [order 2] : [((time == 0) && (PressureSensor))]
  PressurizeCircuit -> Anomaly [order 1] : [((time == 0) && (~PressureSensor))]
  data: PressureSensor input boolean; time local int8 [0..9]; GeneralValve input boolean; anomaly output boolean

== stateflow chart LGS_allFaultStuffDeleted/Digital Part/Computing module2/RetractionSequence ==
  state CloseGeneralValve
    entry: GeneralValve = false;
    entry: stateNumber =int8(6);
  state Idle
    entry: GeneralValve = false;
    entry: OpenDoorValve = false;
    entry: GearRetractionValve = false;
    entry: CloseDoorValve = false;
    entry: stateNumber = int8(0);
  state stimulateGeneralValve
    entry: GeneralValve = true;
    entry: stateNumber = int8(1);
  state InterruptDetected
    entry: GeneralValve = true;
  state StopStimulatingCloseDoorValve
    entry: CloseDoorValve = false;
    entry: stateNumber = int8(5);
  state StimulateOpenDoorValve
    entry: OpenDoorValve = true;
    entry: CloseDoorValve = false;
    entry: stateNumber = int8(2);
  state Interruption
    entry: GearRetractionValve = false;
  state StopGRVandODVstartCDV
    entry: GearRetractionValve = false;
    entry: OpenDoorValve = false;
    entry: CloseDoorValve = true;
    entry: stateNumber = int8(4);
  state StimulateGearRetractionValve
    entry: GearRetractionValve = true;
    entry: stateNumber = int8(3);
  (default) -> Idle
  CloseGeneralValve -> Idle [order 1] : [(~ExtensionInterruption)]
  InterruptDetected -> CloseGeneralValve [order 5] : [(InterruptStateNo == 1)]
  Idle -> InterruptDetected [order 2] : [((InterruptStateNo ~=0) && (StartRetractionSequence))]
  CloseGeneralValve -> Interruption [order 2] : [(ExtensionInterruption)]
  StopStimulatingCloseDoorValve -> CloseGeneralValve [order 1] : [(~ExtensionInterruption)]
  Idle -> stimulateGeneralValve [order 1] : [((((StartRetractionSequence) && (AllDoorsLockedClosed)) && (AllGearsLockedDown)) && (InterruptStateNo == 0))]
  Interruption -> Idle
  InterruptDetected -> stimulateGeneralValve [order 1] : [(InterruptStateNo == 6)]
  InterruptDetected -> StimulateOpenDoorValve [order 4] : [((InterruptStateNo == 4) || (InterruptStateNo == 5))]
  InterruptDetected -> StopGRVandODVstartCDV [order 2] : [(InterruptStateNo == 2)]
  InterruptDetected -> StimulateGearRetractionValve [order 3] : [(InterruptStateNo == 3)]
  stimulateGeneralValve -> StimulateOpenDoorValve [order 1] : [(~ExtensionInterruption)]
  stimulateGeneralValve -> Interruption [order 2] : [(ExtensionInterruption)]
  StopStimulatingCloseDoorValve -> Interruption [order 2] : [(ExtensionInterruption)]
  StopGRVandODVstartCDV -> StopStimulatingCloseDoorValve [order 1] : [((AllDoorsLockedClosed) && (~ExtensionInterruption))]
  StopGRVandODVstartCDV -> Interruption [order 2] : [(ExtensionInterruption)]
  StimulateOpenDoorValve -> Interruption [order 2] : [(ExtensionInterruption)]
  StimulateGearRetractionValve -> Interruption [order 2] : [(ExtensionInterruption)]
  StimulateOpenDoorValve -> StimulateGearRetractionValve [order 1] : [(((AllDoorsOpened) && (AllShockAbsorbersRelaxed)) && (~ExtensionInterruption))]
  StimulateOpenDoorValve -> StopGRVandODVstartCDV [order 3] : [(((AllDoorsOpened) && (~AllShockAbsorbersRelaxed)) && (~ExtensionInterruption))]
  StimulateGearRetractionValve -> StopGRVandODVstartCDV [order 1] : [((AllGearsLockedUp) && (~ExtensionInterruption))]
  data: StartRetractionSequence input boolean; GeneralValve output boolean; OpenDoorValve output boolean; AllDoorsOpened input boolean; AllDoorsLockedClosed input boolean; AllGearsLockedDown input boolean; AllGearsLockedUp input boolean; CloseDoorValve output boolean; AllShockAbsorbersRelaxed input boolean [0..3]; ExtensionInterruption input boolean; GearRetractionValve output boolean; InterruptStateNo input int8 [0..6]; stateNumber output int8 [0..6]

== stateflow chart LGS_allFaultStuffDeleted/Digital Part/Computing module1/OutgoingSequence ==
  state Idle
    entry: GeneralValve = false;
    entry: OpenDoorValve = false;
    entry: GearExtensionValve = false;
    entry: CloseDoorValve = false;
    entry: stateNumber = int8(0);
  state CloseGeneralValve
    entry: GeneralValve = false;
    entry: stateNumber = int8(6);
  state InterruptDetected
    entry: GeneralValve = true;
  state StopStimulatingCloseDoorValve
    entry: CloseDoorValve = false;
    entry: stateNumber = int8(5);
  state stimulateGeneralValve
    entry: GeneralValve = true;
    entry: stateNumber = int8(1);
  state Interruption
    entry: GearExtensionValve = false;
  state StimulateOpenDoorValve
    entry: OpenDoorValve = true;
    entry: CloseDoorValve = false;
    entry: stateNumber = int8(2);
  state StopGEVandODVstartCDV
    entry: GearExtensionValve = false;
    entry: OpenDoorValve = false;
    entry: CloseDoorValve = true;
    entry: stateNumber = int8(4);
  state StimulateGearExtensionValve
    entry: GearExtensionValve = true;
    entry: stateNumber = int8(3);
  (default) -> Idle
  CloseGeneralValve -> Idle [order 1] : [(~RetractionInterruption)]
  InterruptDetected -> CloseGeneralValve [order 2] : [(InterruptStateNo == 1)]
  Idle -> InterruptDetected [order 2] : [((InterruptStateNo ~=0) && (StartOutgoingSequence))]
  CloseGeneralValve -> Interruption [order 2] : [(RetractionInterruption)]
  Interruption -> Idle
  StopStimulatingCloseDoorValve -> CloseGeneralValve [order 1] : [(~RetractionInterruption)]
  Idle -> stimulateGeneralValve [order 1] : [((((StartOutgoingSequence) && (AllGearsLockedUp)) && (AllDoorsLockedClosed)) && (InterruptStateNo == 0))]
  InterruptDetected -> stimulateGeneralValve [order 4] : [(InterruptStateNo == 6)]
  InterruptDetected -> StimulateOpenDoorValve [order 5] : [((InterruptStateNo == 4) || (InterruptStateNo == 5))]
  InterruptDetected -> StopGEVandODVstartCDV [order 3] : [(InterruptStateNo == 2)]
  stimulateGeneralValve -> Interruption [order 1] : [(RetractionInterruption)]
  InterruptDetected -> StimulateGearExtensionValve [order 1] : [(InterruptStateNo == 3)]
  stimulateGeneralValve -> StimulateOpenDoorValve [order 2] : [(~RetractionInterruption)]
  StopStimulatingCloseDoorValve -> Interruption [order 2] : [(RetractionInterruption)]
  StopGEVandODVstartCDV -> StopStimulatingCloseDoorValve [order 1] : [((AllDoorsLockedClosed) && (~RetractionInterruption))]
  StimulateOpenDoorValve -> Interruption [order 2] : [(RetractionInterruption)]
  StimulateGearExtensionValve -> Interruption [order 2] : [(RetractionInterruption)]
  StopGEVandODVstartCDV -> Interruption [order 2] : [(RetractionInterruption)]
  StimulateOpenDoorValve -> StimulateGearExtensionValve [order 1] : [((AllDoorsOpened) && (~RetractionInterruption))]
  StimulateGearExtensionValve -> StopGEVandODVstartCDV [order 1] : [((AllGearsLockedDown) && (~RetractionInterruption))]
  data: StartOutgoingSequence input boolean; GeneralValve output boolean; OpenDoorValve output boolean; AllDoorsOpened input boolean; AllDoorsLockedClosed input boolean; AllGearsLockedDown input boolean; CloseDoorValve output boolean; GearExtensionValve output boolean; AllGearsLockedUp input boolean; stateNumber output int8 [0..6]; RetractionInterruption input boolean; InterruptStateNo input int8 [0..6]

== stateflow chart LGS_allFaultStuffDeleted/Digital Part/Computing module1/PressureSensorMonitoring ==
  state Idle
    entry: anomaly = false;
  state UnpressurizeCircuit
    entry: time = int8(9);
    during: time = time -1;
  note: If the hydraulic circuit is still pressurized 10 seconds after the general electrovalve has been stopped, then an anomaly is detected in the hydraulic circuit.
  state CounterOrder1
  state PressurizeCircuit
    entry: time = int8(1);
    during: time = time - 1;
  state CounterOrder0
  state CircuitPressurized
  note: If the hydraulic circuit is still unpressurized 2 seconds after the general electro-valve has been stimulated, then an anomaly is detected in the hydraulic circuit.
  state Anomaly
    entry: anomaly = true;
  (default) -> Idle
  UnpressurizeCircuit -> Idle [order 2] : [((time == 0) && (~PressureSensor))]
  Idle -> PressurizeCircuit : [(GeneralValve)]
  UnpressurizeCircuit -> CounterOrder1 [order 3] : [(GeneralValve)]
  CounterOrder1 -> PressurizeCircuit
  CounterOrder0 -> UnpressurizeCircuit
  CircuitPressurized -> UnpressurizeCircuit : [(~GeneralValve)]
  UnpressurizeCircuit -> Anomaly [order 1] : [((time == 0) && (PressureSensor))]
  PressurizeCircuit -> CounterOrder0 [order 3] : [(~GeneralValve)]
  PressurizeCircuit -> CircuitPressurized [order 2] : [((time == 0) && (PressureSensor))]
  PressurizeCircuit -> Anomaly [order 1] : [((time == 0) && (~PressureSensor))]
  data: PressureSensor input boolean; time local int8 [0..9]; GeneralValve input boolean; anomaly output boolean
